simulink model "TST_ArraySelectors"  (Simulink 10.0)
settings: Solver=FixedStepDiscrete  StartTime=0.0  StopTime=10.0  FixedStep=0.02  RelTol=1e-3  EnableMultiTasking=on
settings Model: Creator=kharthforeign  LastModifiedBy=unknown
settings DataIOCC: LimitDataPoints=on  SignalLoggingSaveFormat=ModelDataLogs  SaveOutput=off  SignalLogging=off  SaveTime=off
settings OptimizationCC: BlockReduction=off  ConditionallyExecuteInputs=off  OptimizeBlockIOStorage=off  BufferReuse=off  GlobalBufferReuse=off  ExpressionFolding=off  ExpressionDepthLimit=2147483647  LocalBlockOutputs=off  InitFltsAndDblsToZero=on  OptimizeDataStoreBuffers=off  BusAssignmentInplaceUpdate=off
settings DebuggingCC: SolverPrmCheckMsg=warning  FcnCallInpInsideContextMsg=warning  StateNameClashWarn=warning
settings SFSimCC: SimParseCustomCode=off
settings GRTTargetCC: GeneratePreprocessorConditionals=Disable all
settings ConfigComp: CovExternalEMLEnable=off

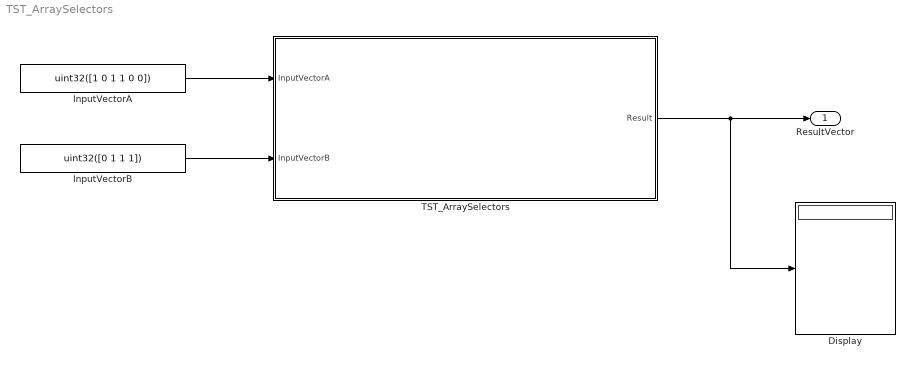
== system TST_ArraySelectors ==
  Display : Display
  InputVectorA : Constant  Value=uint32([1 0 1 1 0 0])
  InputVectorB : Constant  Value=uint32([0 1 1 1])
  TST_ArraySelectors : Subsystem  TreatAsAtomicUnit=on
  ResultVector : Outport
  wires:
  TST_ArraySelectors/1(Result) -> ResultVector/1, Display/1
  InputVectorA/1 -> TST_ArraySelectors/1(InputVectorA)
  InputVectorB/1 -> TST_ArraySelectors/2(InputVectorB)

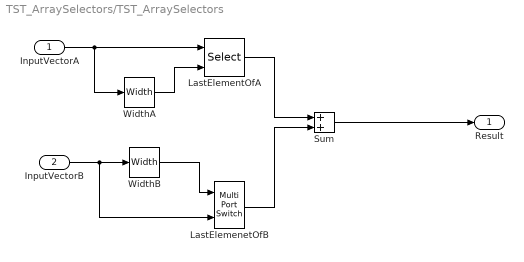
== system TST_ArraySelectors/TST_ArraySelectors ==
  InputVectorA : Inport
  InputVectorB : Inport  Port=2
  LastElemenetOfB : MultiPortSwitch  Inputs=1
  LastElementOfA : Selector  IndexOptions=Index vector (port)  Indices=[1 3]  OutputSizes=1
  Sum : Sum
  WidthA : Width
  WidthB : Width
  Result : Outport
  wires:
  Sum/1 -> Result/1
  InputVectorA/1 -> WidthA/1, LastElementOfA/1
  WidthA/1 -> LastElementOfA/2
  InputVectorB/1 -> WidthB/1, LastElemenetOfB/2
  WidthB/1 -> LastElemenetOfB/1
  LastElementOfA/1 -> Sum/1
  LastElemenetOfB/1 -> Sum/2
